simulink model "motor_param_test"  (Simulink 9.0)
settings: Solver=ode3  StartTime=0.0  StopTime=inf  FixedStep=0.001  RelTol=1e-3  EnableMultiTasking=on
libraries: slrtlib x5, xpcquanserlib x5
settings Model: Creator=Ninad  LastModifiedBy=Joshua  SimulationMode=external
settings DataIOCC: LimitDataPoints=on  SignalLoggingSaveFormat=ModelDataLogs
settings OptimizationCC: BlockReduction=off  OptimizeBlockIOStorage=off  BufferReuse=off  GlobalBufferReuse=off  ExpressionFolding=off  ExpressionDepthLimit=2147483647  LocalBlockOutputs=off
settings DebuggingCC: SolverPrmCheckMsg=warning  FcnCallInpInsideContextMsg=warning  StateNameClashWarn=warning  StrictBusMsg=Warning
settings HardwareCC: ProdIntDivRoundTo=Zero  ProdEndianess=LittleEndian  ProdLongLongMode=on  ProdHWDeviceType=Generic->32-bit x86 compatible
settings RTWCC: SystemTargetFile=slrt.tlc  TemplateMakefile=slrt_default_tmf  Description=Simulink Real-Time  CodeExecutionProfiling=on  RTWCompilerOptimization=on
settings SimulinkRealTimeCC: GeneratePreprocessorConditionals=Disable all
settings ConfigComp: CovSFcnEnable=off

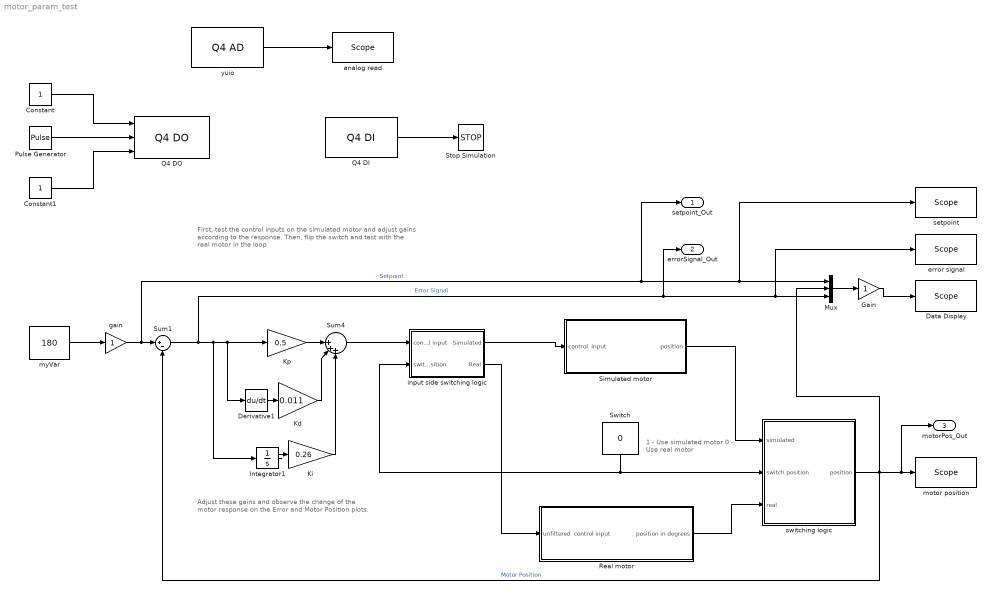
== system motor_param_test ==
  note: Adjust these gains and observe the change of the
      | motor response on the Error and Motor Position
      | plots.
  note: First, test the control inputs on the simulated motor and
      | adjust gains according to the response. Then, flip the switch and
      | test with the real motor in the loop
  note: 1 - Use simulated motor
      | 0 - Use real motor
  Constant : Constant
  Constant1 : Constant
  Data Display : slrtlib/Displays and Logging/Scope   scopeno=3  scopetype=Target  autostart=on  viewmode=Numerical  formatstr="'Setpoint        %3.2f,Motor Position  %3.2f,Error Signal    %3.2f'"  grid=on  ylimits=[0,170]  nosamples=200  noprepostsamples=0  interleave=10  triggermode=FreeRun  triggersignal=1  trigsignalfromport=off  triggerlevel=0.0  triggerslope=Either  triggerscope=1  triggersample=0  filename=data.dat  mode=Lazy  writesize=512  autorestart=off  dynamicfilemode=off  maxwritefilesize=512*1024^2
  Derivative1 : Derivative
  Gain : Gain
  Integrator1 : Integrator
  Kd : Gain  Gain=0.011
  Ki : Gain  Gain=0.26
  Kp : Gain  Gain=0.5
  Mux : Mux  Inputs=3
  Pulse Generator : DiscretePulseGenerator  PulseType=Time based  Period=0.01  PulseWidth=50
  "Q4 DI " : xpcquanserlib/Digital Input/Q4 DI   channel=7  sampleTime=0.001  slot=-1
      settings: SourceProductName=Simulink Real-Time  SourceProductBaseCode=XP
  "Q4 DO " : xpcquanserlib/Digital Output/Q4 DO   channel=[8 6 5]  reset=[1]  initValue=[0]  sampleTime=.001  slot=-1
      settings: SourceProductName=Simulink Real-Time  SourceProductBaseCode=XP
  Real motor : Subsystem
  Simulated motor : Subsystem
  Stop Simulation : Stop
  Sum1 : Sum  Inputs=|+-
  Sum4 : Sum  Inputs=||+++
  Switch : Constant  Value=0
  "analog read " : slrtlib/Displays and Logging/Scope   scopeno=4  scopetype=Target  autostart=on  viewmode=Graphical rolling  formatstr='%15.6f'  grid=on  ylimits=[-1 6]  nosamples=500  noprepostsamples=0  interleave=10  triggermode=FreeRun  triggersignal=1  trigsignalfromport=off  triggerlevel=0.0  triggerslope=Either  triggerscope=1  triggersample=0  filename=data.dat  mode=Lazy  writesize=512  autorestart=off  dynamicfilemode=off  maxwritefilesize=512*1024^2
  error signal : slrtlib/Displays and Logging/Scope   scopeno=2  scopetype=Target  autostart=on  viewmode=Graphical rolling  formatstr='%15.6f'  grid=on  ylimits=[-180,180]  nosamples=500  noprepostsamples=0  interleave=10  triggermode=FreeRun  triggersignal=1  trigsignalfromport=off  triggerlevel=0.0  triggerslope=Either  triggerscope=1  triggersample=0  filename=data.dat  mode=Lazy  writesize=512  autorestart=off  dynamicfilemode=off  maxwritefilesize=512*1024^2
  gain : Gain
  input side switching logic : Subsystem
  motor position : slrtlib/Displays and Logging/Scope   scopeno=7  scopetype=Target  autostart=on  viewmode=Graphical rolling  formatstr='%15.6f'  grid=on  ylimits=[-180,180]  nosamples=500  noprepostsamples=0  interleave=10  triggermode=FreeRun  triggersignal=1  trigsignalfromport=off  triggerlevel=0.0  triggerslope=Either  triggerscope=1  triggersample=0  filename=data.dat  mode=Lazy  writesize=512  autorestart=off  dynamicfilemode=off  maxwritefilesize=512*1024^2
  myVar : Constant  Value=180  OutDataTypeStr=double
  setpoint : slrtlib/Displays and Logging/Scope   scopeno=1  scopetype=Target  autostart=on  viewmode=Graphical rolling  formatstr='%15.6f'  grid=on  ylimits=[-180,180]  nosamples=500  noprepostsamples=0  interleave=10  triggermode=FreeRun  triggersignal=1  trigsignalfromport=off  triggerlevel=0.0  triggerslope=Either  triggerscope=1  triggersample=0  filename=data.dat  mode=Lazy  writesize=512  autorestart=off  dynamicfilemode=off  maxwritefilesize=512*1024^2
  switching logic : Subsystem
  yuio : xpcquanserlib/A//D/Q4 AD  channel=3  sampleTime=0.001  slot=-1
      settings: SourceProductName=Simulink Real-Time  SourceProductBaseCode=XP
  setpoint_Out : Outport
  errorSignal_Out : Outport  Port=2
  motorPos_Out : Outport  Port=3
  wires:
  Kp/1 -> Sum4/1
  Kd/1 -> Sum4/2
  Derivative1/1 -> Kd/1
  Integrator1/1 -> Ki/1
  Ki/1 -> Sum4/3
  gain/1 -> Sum1/1, Mux/1, setpoint/1, setpoint_Out/1  "Setpoint"
  input side switching logic/1(Simulated) -> Simulated motor/1(control  input)
  input side switching logic/2(Real) -> Real motor/1(unfiltered  control input)
  Simulated motor/1(position) -> switching logic/1(simulated)
  Real motor/1(position in degrees) -> switching logic/3(real)
  switching logic/1(position) -> Mux/2, Sum1/2, motor position/1, motorPos_Out/1  "Motor Position"
  Sum4/1 -> input side switching logic/1(control input)
  Switch/1 -> input side switching logic/2(switch  position), switching logic/2(switch position)
  Gain/1 -> Data Display/1
  Mux/1 -> Gain/1
  Sum1/1 -> Kp/1, Derivative1/1, Integrator1/1, Mux/3, error signal/1, errorSignal_Out/1  "Error Signal"
  myVar/1 -> gain/1
  Constant/1 -> "Q4 DO "/1
  "Q4 DI "/1 -> Stop Simulation/1
  yuio/1 -> "analog read "/1
  Pulse Generator/1 -> "Q4 DO "/2
  Constant1/1 -> "Q4 DO "/3

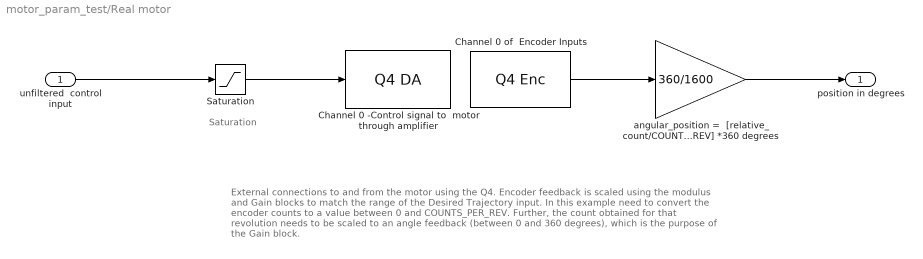
== system motor_param_test/Real motor ==
  note: Saturation
  note: External connections to and from the motor using the Q4.
      |
      | Encoder feedback is scaled using the modulus and Gain blocks to
      | match the range of the Desired Trajectory input.
      |
      | In this example need to convert the encoder counts to a value between 0 and COUNTS_PER_REV.
      | Further, the count obtained for that revolution needs to be scaled to an angle feedback (between
      | 0 and 360 degrees), which is the purpose of the Gain block.
  unfiltered  control input : Inport
  "Channel 0 -Control signal to  motor through amplifier " : xpcquanserlib/D//A/Q4 DA   channel=[1]  range=[-10]  simul=off  reset=[1]  initValue=[0]  sampleTime=.001  slot=-1
      settings: SourceProductName=Simulink Real-Time  SourceProductBaseCode=XP
  "Channel 0 of  Encoder Inputs " : xpcquanserlib/Incremental Encoder/Q4 Enc   channel=2  initialCount=[0]  prescale=[1]  quadrature=[4]  mode=[0]  synchronousIndex=[0]  indexPolarity=[0]  preserveCounts=[0]  sampleTime=.001  slot=-1
      settings: SourceProductName=Simulink Real-Time  SourceProductBaseCode=XP
  Saturation : Saturate  UpperLimit=10  LowerLimit=-10
  angular_position =  [relative_count/COUNTS_PER_REV] *360 degrees : Gain  Gain=360/1600
  position in degrees : Outport
  wires:
  Saturation/1 -> "Channel 0 -Control signal to  motor through amplifier "/1
  angular_position =  [relative_count/COUNTS_PER_REV] *360 degrees/1 -> position in degrees/1
  "Channel 0 of  Encoder Inputs "/1 -> angular_position =  [relative_count/COUNTS_PER_REV] *360 degrees/1
  unfiltered  control input/1 -> Saturation/1

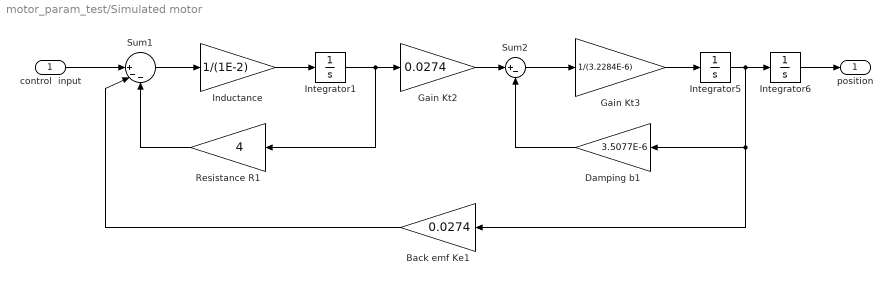
== system motor_param_test/Simulated motor ==
  control  input : Inport
  Back emf Ke1 : Gain  Gain=0.0274
  Damping b1 : Gain  Gain=3.5077E-6
  Gain Kt2 : Gain  Gain=0.0274
  Gain Kt3 : Gain  Gain=1/(3.2284E-6)
  Inductance : Gain  Gain=1/(1E-2)
  Integrator1 : Integrator
  Integrator5 : Integrator
  Integrator6 : Integrator
  Resistance R1 : Gain  Gain=4
  Sum1 : Sum  Inputs=||+--
  Sum2 : Sum  Inputs=|+-
  position : Outport
  wires:
  Sum1/1 -> Inductance/1
  Inductance/1 -> Integrator1/1
  Integrator1/1 -> Gain Kt2/1, Resistance R1/1
  Gain Kt2/1 -> Sum2/1
  Sum2/1 -> Gain Kt3/1
  Gain Kt3/1 -> Integrator5/1
  Integrator5/1 -> Integrator6/1, Back emf Ke1/1, Damping b1/1
  Back emf Ke1/1 -> Sum1/2
  Damping b1/1 -> Sum2/2
  Resistance R1/1 -> Sum1/3
  Integrator6/1 -> position/1
  control  input/1 -> Sum1/1

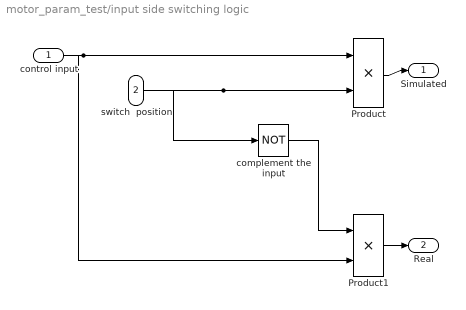
== system motor_param_test/input side switching logic ==
  control input : Inport
  switch  position : Inport  Port=2
  Product : Product  RndMeth=Zero
  Product1 : Product  RndMeth=Zero
  complement the input : Logic  Operator=NOT  AllPortsSameDT=off  OutDataTypeStr=boolean
  Simulated : Outport
  Real : Outport  Port=2
  wires:
  control input/1 -> Product1/2, Product/1
  complement the input/1 -> Product1/1
  switch  position/1 -> complement the input/1, Product/2
  Product/1 -> Simulated/1
  Product1/1 -> Real/1

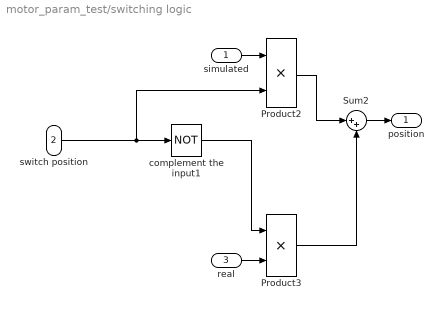
== system motor_param_test/switching logic ==
  simulated : Inport
  switch position : Inport  Port=2
  real : Inport  Port=3
  Product2 : Product  RndMeth=Zero
  Product3 : Product  RndMeth=Zero
  Sum2 : Sum  Inputs=|++
  complement the input1 : Logic  Operator=NOT  AllPortsSameDT=off  OutDataTypeStr=boolean
  position : Outport
  wires:
  complement the input1/1 -> Product3/1
  Product2/1 -> Sum2/1
  Product3/1 -> Sum2/2
  switch position/1 -> Product2/2, complement the input1/1
  simulated/1 -> Product2/1
  Sum2/1 -> position/1
  real/1 -> Product3/2
